simulink model "BeatDetection"  (R2015b)
settings: Solver=ode45  StartTime=0.0  StopTime=inf  RelTol=1e-3
undefined symbols (not defined in the file): dfilt, fdesignblkfcn, gcbh
libraries: simulink x13, dspmtrx3 x4, dsparch4 x3, dspvision x2, dspsnks4 x2, dspswit3 x1, dspxfrm3 x1, dspsigops x1
settings Model: Creator=Hegman  LastModifiedBy=Hegman
settings DataIOCC: SaveFormat=Array
settings DebuggingCC: SolverPrmCheckMsg=warning
settings HardwareCC: ProdBitPerPointer=32  ProdLargestAtomicFloat=None  ProdIntDivRoundTo=Undefined  ProdEndianess=Unspecified  ProdWordSize=32  ProdHWDeviceType=32-bit Generic
settings GRTTargetCC: GeneratePreprocessorConditionals=Disable all
settings ConfigComp: CovModelRefEnable=Off  CovSFcnEnable=off

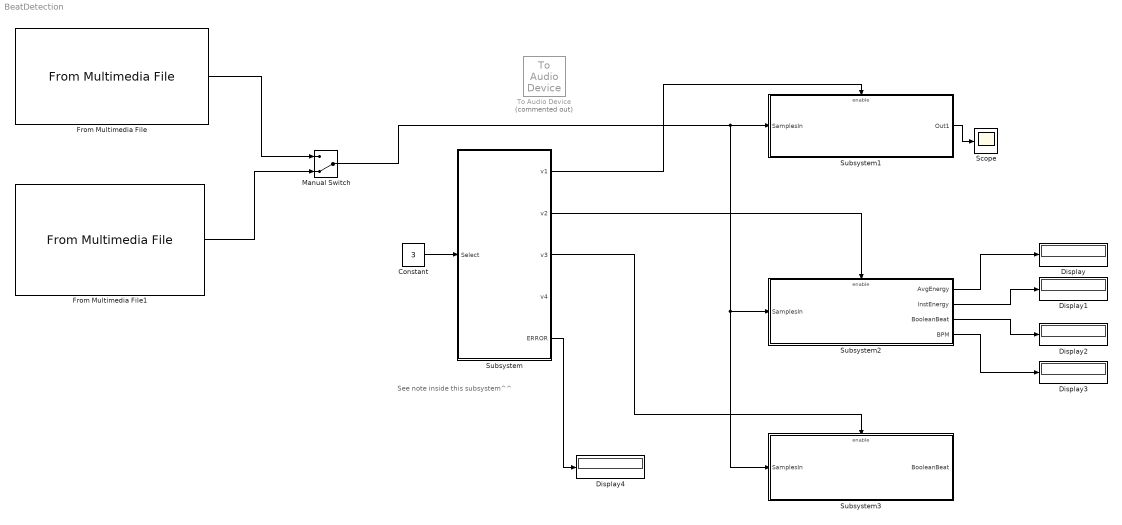
== system BeatDetection ==
  note: See note inside this subsystem^^
  Constant : Constant  Value=3
  Display{,1..4} (5 alike) : Display
  From Multimedia File : dspvision/From Multimedia File  inputFilename=C:\Users\Hegman\Desktop\bass.mp3  loop=on  numPlays=inf  outputStreams=Audio only  videoDataType=single  audioDataType=double  inheritSampleTime=on  userDefinedSampleTime=1/30  noAudioOutput=off  isIntensityVideo=off  fourcc=RGB  colorVideoFormat=Separate color signals  outputEOF=off  dataOrg=Column-major  audioFrameSize=1024  computeAudioFrameSize=off  outSamplingMode=Sample based
  From Multimedia File1 : dspvision/From Multimedia File  inputFilename=C:\Users\Hegman\Desktop\song.mp3  loop=on  numPlays=inf  outputStreams=Audio only  videoDataType=single  audioDataType=double  inheritSampleTime=on  userDefinedSampleTime=1/44  noAudioOutput=off  isIntensityVideo=off  fourcc=RGB  colorVideoFormat=Separate color signals  outputEOF=off  dataOrg=Column-major  audioFrameSize=1024  computeAudioFrameSize=off  outSamplingMode=Sample based
  Manual Switch : ManualSwitch  CurrentSetting=0
  Scope : Scope
  Subsystem : Subsystem
  Subsystem1 : Subsystem
  Subsystem2 : Subsystem
  Subsystem3 : Subsystem
  To Audio Device : dspsnks4/To Audio Device  Commented=on  deviceName=Default  inheritSampleRate=on  sampleRate=45056  deviceDatatype=Determine from input data type  autoBufferSize=on  bufferSize=4096  queueDuration=1.0  defaultOutputChannelMapping=on  outputChannelMapping=1:2  outputNumUnderrunSamples=off
  wires:
  Subsystem1/1(Out1) -> Scope/1
  Subsystem2/1(AvgEnergy) -> Display/1
  Subsystem2/2(InstEnergy) -> Display1/1
  Subsystem2/3(BooleanBeat) -> Display2/1
  Subsystem2/4(BPM) -> Display3/1
  Subsystem/1(v1) -> Subsystem1/Enable
  Subsystem/2(v2) -> Subsystem2/Enable
  Constant/1 -> Subsystem/1(Select)
  Subsystem/3(v3) -> Subsystem3/Enable
  Subsystem/5(ERROR) -> Display4/1
  From Multimedia File/1 -> Manual Switch/1
  From Multimedia File1/1 -> Manual Switch/2
  Manual Switch/1 -> Subsystem2/1(SamplesIn), Subsystem3/1(SamplesIn), Subsystem1/1(SamplesIn)

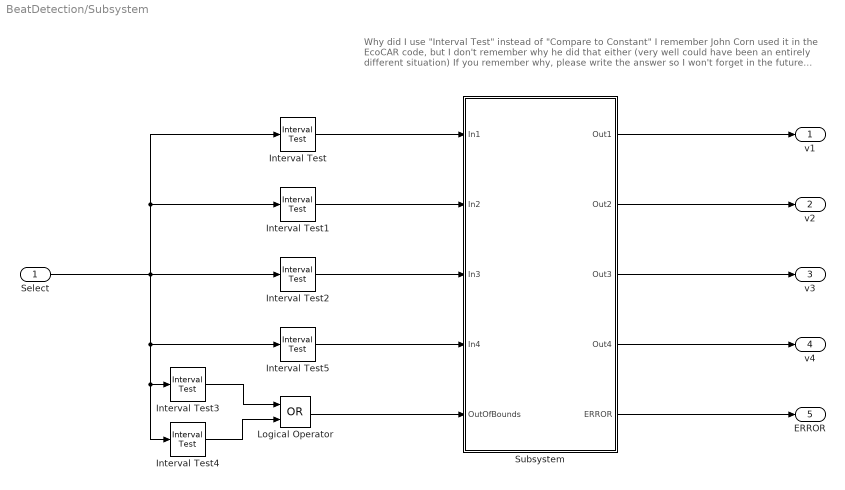
== system BeatDetection/Subsystem ==
  note: Why did I use "Interval Test" instead of "Compare to Constant"
      | I remember John Corn used it in the EcoCAR code, but I don't remember why he did that either (very well could have been an entirely different situation)
      | If you remember why, please write the answer so I won't forget in the future...
  Select : Inport
  Interval Test : simulink/Logic and Bit Operations/Interval Test  IntervalClosedRight=on  uplimit=1  IntervalClosedLeft=on  lowlimit=1  OutDataTypeStr=uint8
  Interval Test1 : simulink/Logic and Bit Operations/Interval Test  IntervalClosedRight=on  uplimit=2  IntervalClosedLeft=on  lowlimit=2  OutDataTypeStr=uint8
  Interval Test2 : simulink/Logic and Bit Operations/Interval Test  IntervalClosedRight=on  uplimit=3  IntervalClosedLeft=on  lowlimit=3  OutDataTypeStr=uint8
  Interval Test3 : simulink/Logic and Bit Operations/Interval Test  IntervalClosedRight=off  uplimit=1  IntervalClosedLeft=on  lowlimit=-inf  OutDataTypeStr=boolean
  Interval Test4 : simulink/Logic and Bit Operations/Interval Test  IntervalClosedRight=on  uplimit=inf  IntervalClosedLeft=off  lowlimit=3  OutDataTypeStr=boolean
  Interval Test5 : simulink/Logic and Bit Operations/Interval Test  IntervalClosedRight=on  uplimit=4  IntervalClosedLeft=on  lowlimit=4  OutDataTypeStr=uint8
  Logical Operator : Logic  Operator=OR  AllPortsSameDT=off
  Subsystem : Subsystem
  v1 : Outport
  v2 : Outport  Port=2
  v3 : Outport  Port=3
  v4 : Outport  Port=4
  ERROR : Outport  Port=5
  wires:
  Interval Test3/1 -> Logical Operator/1
  Interval Test4/1 -> Logical Operator/2
  Select/1 -> Interval Test/1, Interval Test1/1, Interval Test5/1, Interval Test4/1, Interval Test3/1, Interval Test2/1
  Interval Test1/1 -> Subsystem/2(In2)
  Interval Test2/1 -> Subsystem/3(In3)
  Logical Operator/1 -> Subsystem/5(OutOfBounds)
  Interval Test/1 -> Subsystem/1(In1)
  Subsystem/1(Out1) -> v1/1
  Subsystem/2(Out2) -> v2/1
  Subsystem/3(Out3) -> v3/1
  Subsystem/5(ERROR) -> ERROR/1
  Interval Test5/1 -> Subsystem/4(In4)
  Subsystem/4(Out4) -> v4/1

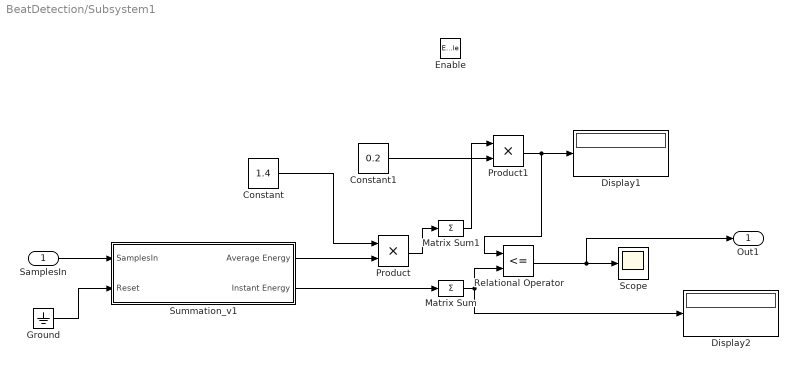
== system BeatDetection/Subsystem1 ==
  SamplesIn : Inport
  Enable : EnablePort
  Constant : Constant  Value=1.4
  Constant1 : Constant  Value=0.2
  Display1 : Display
  Display2 : Display
  Ground : Ground
  Matrix Sum : Sum  Inputs=+
  Matrix Sum1 : Sum  Inputs=+
  Product : Product
  Product1 : Product
  Relational Operator : RelationalOperator  Operator=<=  OutDataTypeStr=boolean
  Scope : Scope
  Summation_v1 : Subsystem
  Out1 : Outport
  wires:
  Summation_v1/1(Average Energy) -> Product/2
  Constant/1 -> Product/1
  Relational Operator/1 -> Out1/1, Scope/1
  Summation_v1/2(Instant Energy) -> Matrix Sum/1
  Matrix Sum/1 -> Display2/1, Relational Operator/2
  Product/1 -> Matrix Sum1/1
  Product1/1 -> Relational Operator/1, Display1/1
  Matrix Sum1/1 -> Product1/1
  Constant1/1 -> Product1/2
  SamplesIn/1 -> Summation_v1/1(SamplesIn)
  Ground/1 -> Summation_v1/2(Reset)

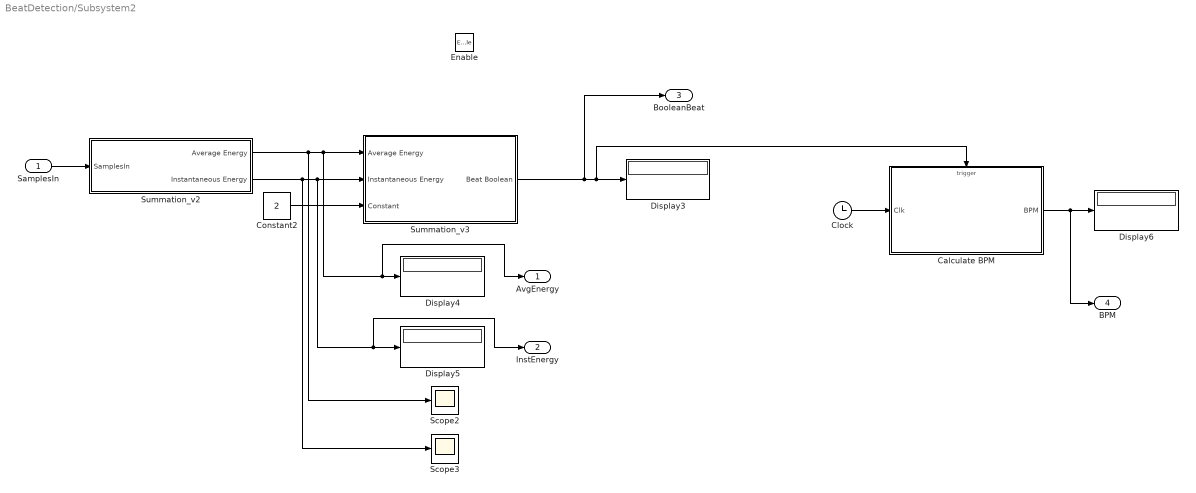
== system BeatDetection/Subsystem2 ==
  SamplesIn : Inport
  Enable : EnablePort
  Calculate BPM : Subsystem
  Clock : Clock
  Constant2 : Constant  Value=2
  Display{3..6} (4 alike) : Display
  Scope2 : Scope
  Scope3 : Scope
  Summation_v2 : Subsystem
  Summation_v3 : Subsystem
  AvgEnergy : Outport
  InstEnergy : Outport  Port=2
  BooleanBeat : Outport  Port=3
  BPM : Outport  Port=4
  wires:
  Summation_v2/1(Average Energy) -> Scope2/1, AvgEnergy/1, Display4/1, Summation_v3/1(Average Energy)
  Summation_v2/2(Instantaneous Energy) -> Scope3/1, InstEnergy/1, Display5/1, Summation_v3/2(Instantaneous Energy)
  Constant2/1 -> Summation_v3/3(Constant)
  Summation_v3/1(Beat Boolean) -> BooleanBeat/1, Calculate BPM/Trigger, Display3/1
  Clock/1 -> Calculate BPM/1(Clk)
  Calculate BPM/1(BPM) -> BPM/1, Display6/1
  SamplesIn/1 -> Summation_v2/1(SamplesIn)

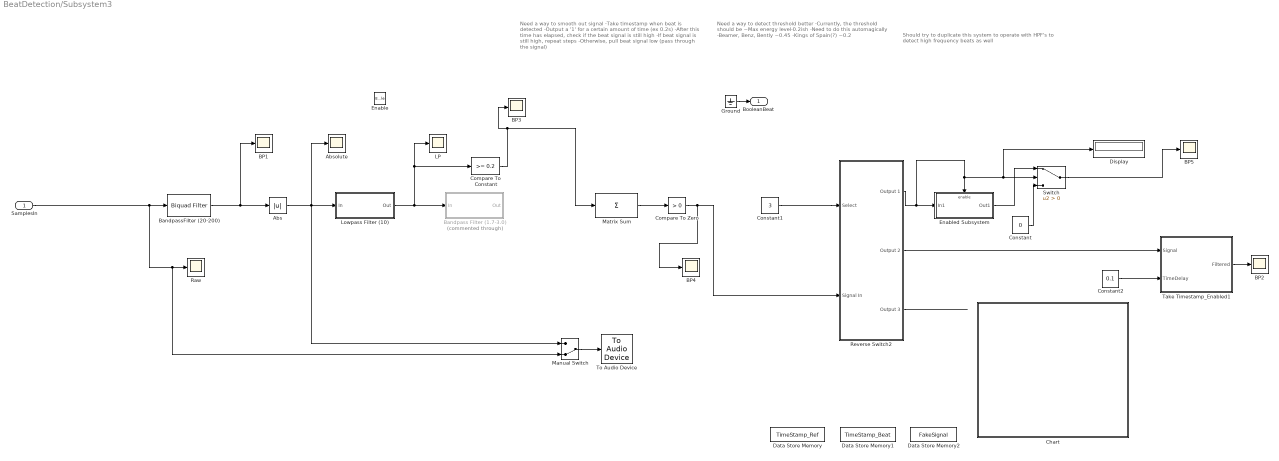
== system BeatDetection/Subsystem3 ==
  note: Need a way to smooth out signal
      | -Take timestamp when beat is detected
      | -Output a '1' for a certain amount of time (ex 0.2s)
      | -After this time has elapsed, check if the beat signal is still high
      | -If beat signal is still high, repeat steps
      | -Otherwise, pull beat signal low (pass through the signal)
  note: Need a way to detect threshold better
      | -Currently, the threshold should be ~Max energy level-0.2ish
      | -Need to do this automagically
      | -Beamer, Benz, Bently ~0.45
      | -Kings of Spain(?) ~0.2
  note: Should try to duplicate this system to operate with HPF's
      | to detect high frequency beats as well
  SamplesIn : Inport
  Enable : EnablePort
  Abs : Abs
  Absolute : Scope
  BP{1..5} (5 alike) : Scope
  Bandpass Filter (1.7-3.0) : Subsystem  Commented=through  DialogController=fdesignblkfcn  InitFcn=fdesignblkfcn(gcbh, {'InitFcn'});  mask(Bandpass Filter){}
      mask help: Design a bandpass filter
      settings: CopyFcn=fdesignblkfcn(gcbh, {'CopyFcn'});
      mask Help: helpview(mapfilelocation('dsp'), 'dspbandpassfilter');
      mask Display: disp('Bandpass');
  BandpassFilter (20-200) : dsparch4/Biquad Filter  Tag=BlockMethodSubSystem  IIRFiltStruct=Direct form II  CoeffSource=Specify via dialog  BiQuadCoeffs=[0.0031095318629756033 0 -0.0031095318629756033 1 -1.9981397557432883 0.99814821478936055;0.13570010317958014 0 -0.13570010317958014 1 -1.9940050318428257 0.9940167705198949;0.089106046740989542 0 -0.089106046740989542 1 -1.9816119239202097 0.98238370304407796;2 0 -2 1 -1.9589067705035481 0.95945538503128502]  a0Flag=Warning  IC=0  ICnum=0  ICden=0  InputProcessing=Columns as channels (frame based)  denAccumFracLength=30  denProdOutputFracLength=30  secondMemoryFracLength=15  roundingMode=Floor  overflowMode=off  ScaleValues=[5.1280917433920097e-06;1;1;1;67.812469673723953]  optimizeScaleValues=on  ScaleValueMode=Specify via input port (g)  scaleValueFracLength=14  FilterSource=Specify via dialog  FilterObject=dfilt.df2tsos([1 0.3 0.4],[1 0.1 0.2])
  Chart : Stateflow chart  TreatAsAtomicUnit=on
  Compare To Constant : simulink/Logic and Bit Operations/Compare To Constant  relop=>=  const=0.2  OutDataTypeStr=boolean
  Compare To Zero : simulink/Logic and Bit Operations/Compare To Zero  relop=>  OutDataTypeStr=uint8
  Constant : Constant  Value=0
  Constant1 : Constant  Value=3
  Constant2 : Constant  Value=0.1
  Data Store Memory : DataStoreMemory  DataStoreName=TimeStamp_Ref  ReadBeforeWriteMsg=warning  WriteAfterWriteMsg=warning  WriteAfterReadMsg=warning
  Data Store Memory1 : DataStoreMemory  DataStoreName=TimeStamp_Beat  ReadBeforeWriteMsg=warning  WriteAfterWriteMsg=warning  WriteAfterReadMsg=warning
  Data Store Memory2 : DataStoreMemory  DataStoreName=FakeSignal  ReadBeforeWriteMsg=warning  WriteAfterWriteMsg=warning  WriteAfterReadMsg=warning
  Display : Display
  Enabled Subsystem : Subsystem  TreatAsAtomicUnit=on
  Ground : Ground
  LP : Scope
  Lowpass Filter (10) : Subsystem  DialogController=fdesignblkfcn  InitFcn=fdesignblkfcn(gcbh, {'InitFcn'});  mask(Lowpass Filter){}
      mask help: Design a lowpass filter
      settings: CopyFcn=fdesignblkfcn(gcbh, {'CopyFcn'});
      mask Help: helpview(mapfilelocation('dsp'), 'dsplowpassfilter');
      mask Display: disp('Lowpass')
  Manual Switch : ManualSwitch  CurrentSetting=0
  Matrix Sum : Sum  Inputs=+
  Raw : Scope
  Reverse Switch2 : Subsystem
  Switch : Switch  Criteria=u2 > Threshold
  Take Timestamp_Enabled1 : Subsystem
  To Audio Device : dspsnks4/To Audio Device  deviceName=Default  inheritSampleRate=on  sampleRate=45056  deviceDatatype=Determine from input data type  autoBufferSize=on  bufferSize=4096  queueDuration=1.0  defaultOutputChannelMapping=on  outputChannelMapping=1:2  outputNumUnderrunSamples=off
  BooleanBeat : Outport
  wires:
  Ground/1 -> BooleanBeat/1
  SamplesIn/1 -> BandpassFilter (20-200)/1, Manual Switch/2, Raw/1
  BandpassFilter (20-200)/1 -> Abs/1, BP1/1
  Manual Switch/1 -> To Audio Device/1
  Abs/1 -> Manual Switch/1, Absolute/1, Lowpass Filter (10)/1(In)
  Lowpass Filter (10)/1(Out) -> Compare To Constant/1, LP/1, Bandpass Filter (1.7-3.0)/1(In)
  Compare To Constant/1 -> BP3/1, Matrix Sum/1
  Matrix Sum/1 -> Compare To Zero/1
  Compare To Zero/1 -> Reverse Switch2/2(Signal In), BP4/1
  Enabled Subsystem/1(Out1) -> Switch/1
  Constant/1 -> Switch/3
  Switch/1 -> BP5/1
  Reverse Switch2/1(Output 1) -> Display/1, Switch/2, Enabled Subsystem/Enable, Enabled Subsystem/1(In1)
  Reverse Switch2/2(Output 2) -> Take Timestamp_Enabled1/1(Signal)
  Constant1/1 -> Reverse Switch2/1(Select)
  Take Timestamp_Enabled1/1(Filtered) -> BP2/1
  Constant2/1 -> Take Timestamp_Enabled1/2(TimeDelay)
  Reverse Switch2/3(Output 3) -> ?

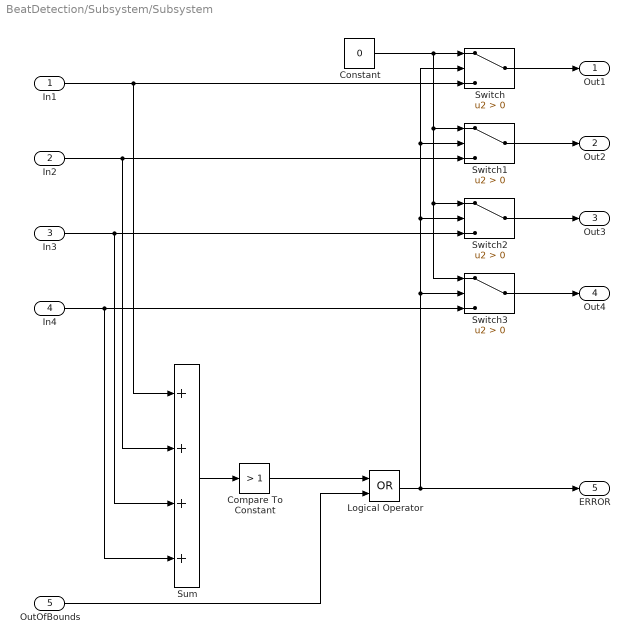
== system BeatDetection/Subsystem/Subsystem ==
  In1 : Inport
  In2 : Inport  Port=2
  In3 : Inport  Port=3
  In4 : Inport  Port=4
  OutOfBounds : Inport  Port=5
  Compare To Constant : simulink/Logic and Bit Operations/Compare To Constant  relop=>  const=1  OutDataTypeStr=boolean
  Constant : Constant  Value=0
  Logical Operator : Logic  Operator=OR  AllPortsSameDT=off  OutDataTypeStr=boolean
  Sum : Sum  Inputs=++++
  Switch{,1..3} (4 alike) : Switch  Criteria=u2 > Threshold
  Out1 : Outport
  Out2 : Outport  Port=2
  Out3 : Outport  Port=3
  Out4 : Outport  Port=4
  ERROR : Outport  Port=5
  wires:
  In1/1 -> Switch/3, Sum/1
  In2/1 -> Switch1/3, Sum/2
  In3/1 -> Switch2/3, Sum/3
  Sum/1 -> Compare To Constant/1
  OutOfBounds/1 -> Logical Operator/2
  Compare To Constant/1 -> Logical Operator/1
  Logical Operator/1 -> Switch3/2, Switch/2, Switch1/2, Switch2/2, ERROR/1
  Switch/1 -> Out1/1
  Switch1/1 -> Out2/1
  Switch2/1 -> Out3/1
  Constant/1 -> Switch2/1, Switch3/1, Switch1/1, Switch/1
  In4/1 -> Sum/4, Switch3/3
  Switch3/1 -> Out4/1

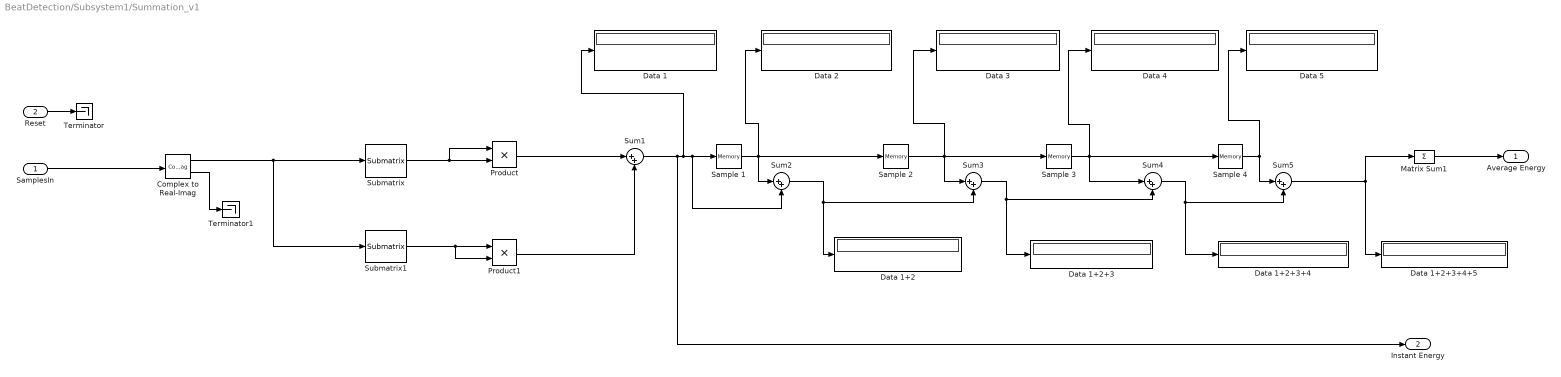
== system BeatDetection/Subsystem1/Summation_v1 ==
  SamplesIn : Inport
  Reset : Inport  Port=2
  Complex to Real-Imag : ComplexToRealImag
  Data {1..5} (5 alike) : Display
  Data 1+2 : Display
  Data 1+2+3 : Display
  Data 1+2+3+4 : Display
  Data 1+2+3+4+5 : Display
  Matrix Sum1 : Sum  Inputs=+
  Product : Product
  Product1 : Product
  Sample {1..4} (4 alike) : Memory
  Submatrix : dspmtrx3/Submatrix  RowSpan=Range of rows  RowStartMode=First  RowStartIndex=1  RowEndMode=Last  RowEndIndex=1  ColSpan=One column  ColStartMode=Index  ColStartIndex=1  ColEndMode=Last  ColEndIndex=1
  Submatrix1 : dspmtrx3/Submatrix  RowSpan=Range of rows  RowStartMode=First  RowStartIndex=1  RowEndMode=Last  RowEndIndex=1  ColSpan=One column  ColStartMode=Index  ColStartIndex=2  ColEndMode=Last  ColEndIndex=1
  Sum{1..5} (5 alike) : Sum  Inputs=|++
  Terminator : Terminator
  Terminator1 : Terminator
  Average Energy : Outport
  Instant Energy : Outport  Port=2
  wires:
  Submatrix1/1 -> Product1/2, Product1/1
  Submatrix/1 -> Product/2, Product/1
  Product/1 -> Sum1/1
  Product1/1 -> Sum1/2
  SamplesIn/1 -> Complex to Real-Imag/1
  Complex to Real-Imag/1 -> Submatrix1/1, Submatrix/1
  Complex to Real-Imag/2 -> Terminator1/1
  Sum1/1 -> Instant Energy/1, Sample 1/1, Sum2/2, Data 1/1
  Sample 1/1 -> Sum2/1, Sample 2/1, Data 2/1
  Sample 2/1 -> Sum3/1, Sample 3/1, Data 3/1
  Sample 3/1 -> Sum4/1, Sample 4/1, Data 4/1
  Sample 4/1 -> Sum5/1, Data 5/1
  Sum2/1 -> Sum3/2, Data 1+2/1
  Sum3/1 -> Sum4/2, Data 1+2+3/1
  Sum4/1 -> Sum5/2, Data 1+2+3+4/1
  Sum5/1 -> Data 1+2+3+4+5/1, Matrix Sum1/1
  Matrix Sum1/1 -> Average Energy/1
  Reset/1 -> Terminator/1

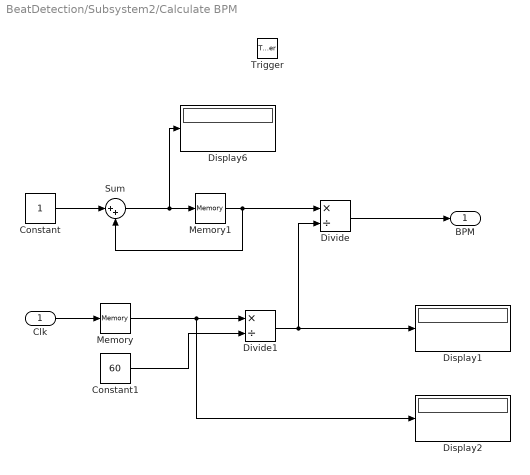
== system BeatDetection/Subsystem2/Calculate BPM ==
  Clk : Inport
  Trigger : TriggerPort  PortDimensions=1
  Constant : Constant
  Constant1 : Constant  Value=60
  Display1 : Display
  Display2 : Display
  Display6 : Display
  Divide : Product  Inputs=*/
  Divide1 : Product  Inputs=*/
  Memory : Memory  InheritSampleTime=on
  Memory1 : Memory  InheritSampleTime=on
  Sum : Sum  Inputs=|++
  BPM : Outport
  wires:
  Constant/1 -> Sum/1
  Sum/1 -> Display6/1, Memory1/1
  Memory1/1 -> Divide/1, Sum/2
  Clk/1 -> Memory/1
  Constant1/1 -> Divide1/2
  Memory/1 -> Display2/1, Divide1/1
  Divide1/1 -> Display1/1, Divide/2
  Divide/1 -> BPM/1

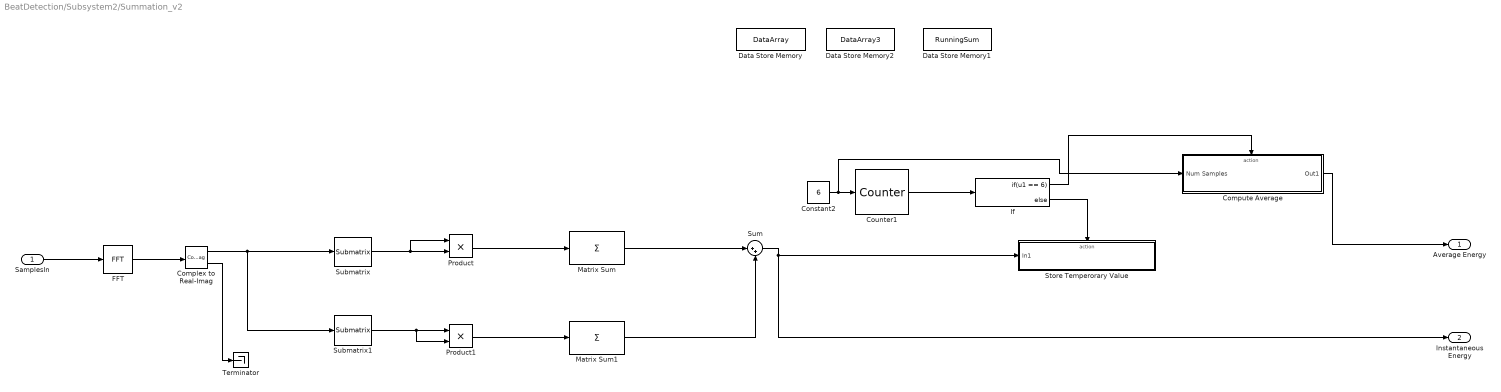
== system BeatDetection/Subsystem2/Summation_v2 ==
  SamplesIn : Inport
  Complex to Real-Imag : ComplexToRealImag
  Compute Average : Subsystem  TreatAsAtomicUnit=on
  Constant2 : Constant  Value=6  OutDataTypeStr=uint8
  Counter1 : dspswit3/Counter  Direction=Up  CountEvent=Free running  CounterSize=Specify via input port  MaxCount=43  InitialCount=0  Output=Count  HitValue=32  ResetInput=off  SamplesPerFrame=1  Ts=0.02321995464852607709750566893424  CntDtype=double  HitDtype=Logical
  Data Store Memory : DataStoreMemory  DataStoreName=DataArray  ReadBeforeWriteMsg=warning  WriteAfterWriteMsg=warning  WriteAfterReadMsg=warning  InitialValue=[0 0 0 0 0 0]
  Data Store Memory1 : DataStoreMemory  DataStoreName=RunningSum  ReadBeforeWriteMsg=warning  WriteAfterWriteMsg=warning  WriteAfterReadMsg=warning
  Data Store Memory2 : DataStoreMemory  DataStoreName=DataArray3  ReadBeforeWriteMsg=warning  WriteAfterWriteMsg=warning  WriteAfterReadMsg=warning  InitialValue=[0 0 0 0 0 0 0 0 0 0 0 0 0 0 0 0 0 0 0 0 0 0 0 0 0 0 0 0 0 0 0 0 0 0 0 0 0 0 0 0 0 0 0 0 0 0 0 0 0 0 0 0 0 0 0 0 0 0 0 0 0 0 0 0 0 0 0 0 0 0 0 0 0 0 0 0 0 0 0 0 0 0 0 0 0 0 0 0 0 0 0 0 0 0 0 0 0 0 0 0 0 0 0 0 0 0 0 0 0 0 0 0 0 0 0 0 0 0 0 0 0 0 0 0 0 0 0 0 0 0 0 0 0 0 0 0 0 0 0 0 0 0 0 0 0 0 0 0 0 0 0 0 0 0 0 0 0 0 0 0 0 0 0 0 0 0 0 0 0 0 0 0 0 0 0 0 0 0 0 0 0 0 0 0 0 0 0 0 0 0 0 0 0 0 0 0 0 0 0 0 0 0 0 0 0 0 0 0 0 0 0 0 0 0 0 0 0 0 0 0 0 0 0 0 0 0 0 0 0 0 0 0 0 0 0 0 0 0 0 0 0 0 0 0 0 0 0 0 0 0 0 0 0 0 0 0 0 0 0 0 0 0 0 0 0 0 0 0 0 0 0 0 0 0 0 0 0 0 0 0 0 0 0 0 0 0 0 0 0 0 0 0 0 0 0 0 0 0 0 0 0 0 0 0 0 0 0 0 0 0 0 0 0 0 0 0 0 0 0 0 0 0 0 0 0 0 0 0 0 0 0 0 0 0 0 0 0 0 0 0 0 0 0 0 0 0 0 0 0 0 0 0 0 0 0 0 0 0 0 0 0 0 0 0 0 0 0 0 0 0 0 0 0 0 0 0 0 0 0 0 0 0 0 0 0 0 0 0 0 0 0 0 0 0 0 0 0 0 0 0 0 0 0 0 0 0 0 0 0 0 0 0 0 0 0 0 0 0 0 0 0 0 0 0 0 0 0 0 0 0 0 0 0 0 0 0 0 0 0 0 0 0 0 0 0 0 0 0 0 0 0 0 0 0 0 0 0 0 0 0 0 0 0 0 0 0 0 0 0 0 0 0 0 0 0 0 0 0 0 0 0 0 0 0 0 0 0 0 0 0 0 0 0 0 0 0 0 0 0 0 0 0 0 0 0 0 0 0 0 0 0 0 0 0 0 0 0 0 0 0 0 0 0 0 0 0 0 0 0 0 0 0 0 0 0 0 0 0 0 0 0 0 0 0 0 0 0 0 0 0 0 0 0 0 0 0 0 0 0 0 0 0 0 0 0 0 0 0 0 0 0 0 0 0 0 0 0 0 0 0 0 0 0 0 0 0 0 0 0 0 0 0 0 0 0 0 0 0 0 0 0 0 0 0 0 0 0 0 0 0 0 0 0 0 0 0 0 0 0 0 0 0 0 0 0 0 0 0 0 0 0 0 0 0 0 0 0 0 0 0 0 0 0 0 0 0 0 0 0 0 0 0 0 0 0 0 0 0 0 0 0 0 0 0 0 0 0 0 0 0 0 0 0 0 0 0 0 0 0 0 0 0 0 0 0 0 0 0 0 0 0 0 0 0 0 0 0 0 0 0 0 0 0 0 0 0 0 0 0 0 0 0 0 0 0 0 0 0 0 0 0 0 0 0 0 0 0 0 0 0 0 0 0 0 0 0 0 0 0 0 0 0 0 0 0 0 0 0 0 0 0 0 0 0 0 0 0 0 0 0 0 0 0 0 0 0 0 0 0 0 0 0 0 0 0 0 0 0 0 0 0 0 0 0 0 0 0 0 0 0 0 0 0 0 0 0 0 0 0 0 0 0 0 0 0 0 0 0 0 0 0 0 0 0 0 0 0 0 0 0 0 0 0 0 0 0 0 0 0 0 0 0 0 0 0 0 0 0 0 0 0 0 0 0 0 0 0 0 0 0 0 0 0 0 0 0 0 0 0 0 0 0 0 0 0 0 0 0 0 0 0 0 0 0 0 0 0 0 0 0 0 0 0 0 0 0 0 0 0 0 0 0 0 0 0 0 0 0 0 0 0 0 0 0 0 0 0 0 0 0 0 0 0 0 0 0 0 0 0 0 0 0 0 0 0 0 0 0 0 0 0 0 0 0 0 0 0 0 0 0 0 0 0 0 0 0 0 0 0 0 0 0 0 0 0 0 0 0 0 0 0 0 0 0 0 0 0 0 0 0 0 0 0 0 0 0 0 0 0 0 0 0 0 0 0 0 0 0 0 0 0 0 0 0 0 0 0 0 0 0 0 0 0 0 0 0 0 0 0 0 0 0 0 0 0 0 0 0 0 0 0 0 0 0]
  FFT : dspxfrm3/FFT  FFTImplementation=Auto  CompMethod=Table lookup  TableOpt=NEW  TableOptActive=Speed  BitRevOrder=off  Normalize=off  InheritFFTLength=on  FFTLength=64  WrapInput=on  roundingMode=Floor  overflowMode=off  firstCoeffDataTypeStr=Inherit: Same word length as input  firstCoeffLastDataTypeStr=Inherit: Same word length as input  outputMin=[]  outputMax=[]
  If : If  IfExpression=u1 == 6
  Matrix Sum : Sum  Inputs=+
  Matrix Sum1 : Sum  Inputs=+
  Product : Product
  Product1 : Product
  Store Temperorary Value : Subsystem  TreatAsAtomicUnit=on
  Submatrix : dspmtrx3/Submatrix  RowSpan=Range of rows  RowStartMode=First  RowStartIndex=1  RowEndMode=Last  RowEndIndex=1  ColSpan=One column  ColStartMode=Index  ColStartIndex=1  ColEndMode=Last  ColEndIndex=1
  Submatrix1 : dspmtrx3/Submatrix  RowSpan=Range of rows  RowStartMode=First  RowStartIndex=1  RowEndMode=Last  RowEndIndex=1  ColSpan=One column  ColStartMode=Index  ColStartIndex=2  ColEndMode=Last  ColEndIndex=1
  Sum : Sum  Inputs=|++
  Terminator : Terminator
  Average Energy : Outport
  Instantaneous Energy : Outport  Port=2
  wires:
  Submatrix1/1 -> Product1/2, Product1/1
  Submatrix/1 -> Product/2, Product/1
  Product/1 -> Matrix Sum/1
  Product1/1 -> Matrix Sum1/1
  Matrix Sum/1 -> Sum/1
  Matrix Sum1/1 -> Sum/2
  Compute Average/1(Out1) -> Average Energy/1
  Constant2/1 -> Compute Average/1(Num Samples), Counter1/1
  Counter1/1 -> If/1
  If/1 -> Compute Average/Action
  Sum/1 -> Instantaneous Energy/1, Store Temperorary Value/1(In1)
  If/2 -> Store Temperorary Value/Action
  SamplesIn/1 -> FFT/1
  FFT/1 -> Complex to Real-Imag/1
  Complex to Real-Imag/1 -> Submatrix1/1, Submatrix/1
  Complex to Real-Imag/2 -> Terminator/1

== system BeatDetection/Subsystem2/Summation_v3 ==
  Average Energy : Inport
  Instantaneous Energy : Inport  Port=2
  Constant : Inport  Port=3
  Product : Product
  Relational Operator : RelationalOperator  Operator=<=  OutDataTypeStr=boolean
  Beat Boolean : Outport
  wires:
  Average Energy/1 -> Product/1
  Constant/1 -> Product/2
  Product/1 -> Relational Operator/1
  Instantaneous Energy/1 -> Relational Operator/2
  Relational Operator/1 -> Beat Boolean/1

== system BeatDetection/Subsystem3/Bandpass Filter (1.7-3.0) ==
  In : Inport
  Generated Filter Block : dsparch4/Biquad Filter  Tag=BlockMethodSubSystem  IIRFiltStruct=Direct form II  CoeffSource=Specify via dialog  BiQuadCoeffs=[5.4972901029509049e-05 0 -5.4972901029509049e-05 1 -1.9999520618723361 0.99995213446416487;0.00014448691002993394 0 -0.00014448691002993394 1 -1.9999059466356592 0.99990611089951908;9.0735971124424031e-05 0 -9.0735971124424031e-05 1 -1.999837449546598 0.99983750496372492;2 0 -2 1 -1.9998201282991981 0.99982028501520182]  a0Flag=Warning  IC=0  ICnum=0  ICden=0  InputProcessing=Columns as channels (frame based)  denAccumFracLength=30  denProdOutputFracLength=30  secondMemoryFracLength=15  roundingMode=Floor  overflowMode=off  ScaleValues=[7.259182877028536e-08;1;1;1;702.81183193528454]  optimizeScaleValues=off  ScaleValueMode=Specify via input port (g)  scaleValueFracLength=14  FilterSource=Specify via dialog  dfiltObjectName=dfilt.df2tsos([1 0.3 0.4],[1 0.1 0.2])
  Out : Outport
  wires:
  In/1 -> Generated Filter Block/1
  Generated Filter Block/1 -> Out/1

== system BeatDetection/Subsystem3/Enabled Subsystem ==
  In1 : Inport
  Enable : EnablePort
  Pulse Generator : DiscretePulseGenerator  PulseType=Time based  Period=0.4  PulseWidth=50
  Sample and Hold1 : dspsigops/Sample and Hold  trig=Either edge  initCond=0  latchinput=off
  Out1 : Outport
  wires:
  Sample and Hold1/1 -> Out1/1
  In1/1 -> Sample and Hold1/1
  Pulse Generator/1 -> Sample and Hold1/Trigger

== system BeatDetection/Subsystem3/Lowpass Filter (10) ==
  In : Inport
  Generated Filter Block : dsparch4/Biquad Filter  Tag=BlockMethodSubSystem  IIRFiltStruct=Direct form II  CoeffSource=Specify via dialog  BiQuadCoeffs=[3.3035044053868198e-07 6.6070088107736397e-07 3.3035044053868198e-07 1 -1.9976314897873875 0.99763351732213079;7.7829268025137561e-07 1.5565853605027512e-06 7.7829268025137561e-07 1 -1.9994422120745921 0.99944424144716315;5.0708276040372059e-07 1.0141655208074412e-06 5.0708276040372059e-07 1 -1.9972071092702939 0.99720913637430386;0.25000000910851183 0.50000001821702367 0.25000000910851183 1 -1.9984161174213928 0.99841814575250887]  a0Flag=Warning  IC=0  ICnum=0  ICden=0  InputProcessing=Columns as channels (frame based)  denAccumFracLength=30  denProdOutputFracLength=30  secondMemoryFracLength=15  roundingMode=Floor  overflowMode=off  ScaleValues=[2.0275347434317585e-06;1;1;1;1]  optimizeScaleValues=off  ScaleValueMode=Specify via input port (g)  scaleValueFracLength=14  FilterSource=Specify via dialog  FilterObject=dfilt.df2tsos([1 0.3 0.4],[1 0.1 0.2])
  Out : Outport
  wires:
  In/1 -> Generated Filter Block/1
  Generated Filter Block/1 -> Out/1

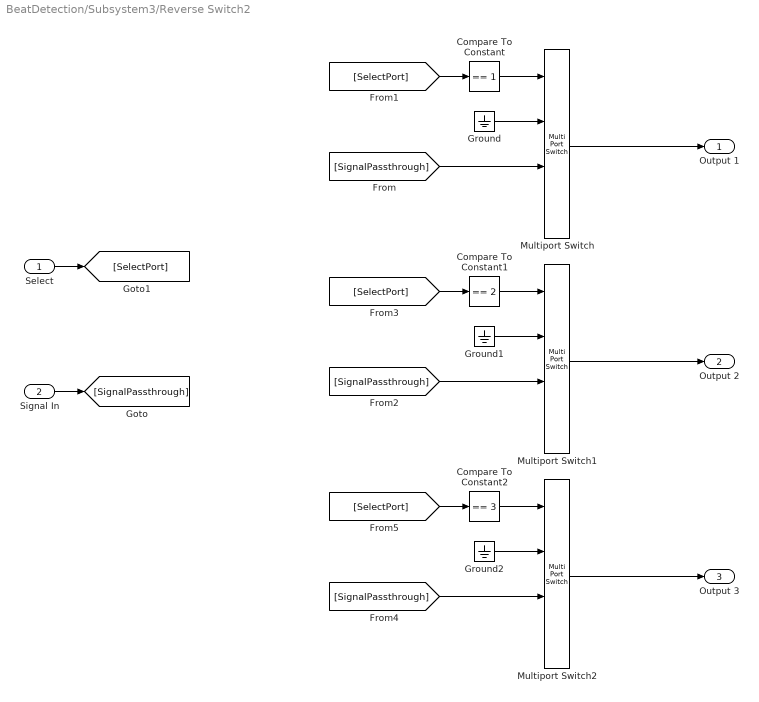
== system BeatDetection/Subsystem3/Reverse Switch2 ==
  Select : Inport
  Signal In : Inport  Port=2
  Compare To Constant : simulink/Logic and Bit Operations/Compare To Constant  relop===  const=1  OutDataTypeStr=uint8
  Compare To Constant1 : simulink/Logic and Bit Operations/Compare To Constant  relop===  const=2  OutDataTypeStr=uint8
  Compare To Constant2 : simulink/Logic and Bit Operations/Compare To Constant  relop===  const=3  OutDataTypeStr=uint8
  Ground : Ground
  Ground1 : Ground
  Ground2 : Ground
  Multiport Switch : MultiPortSwitch  DataPortOrder=Zero-based contiguous  Inputs=2  DataPortForDefault=Additional data port
  Multiport Switch1 : MultiPortSwitch  DataPortOrder=Zero-based contiguous  Inputs=2  DataPortForDefault=Additional data port
  Multiport Switch2 : MultiPortSwitch  DataPortOrder=Zero-based contiguous  Inputs=2  DataPortForDefault=Additional data port
  Output 1 : Outport
  Output 2 : Outport  Port=2
  Output 3 : Outport  Port=3
  wires:
  Compare To Constant/1 -> Multiport Switch/1
  Ground/1 -> Multiport Switch/2
  [SignalPassthrough] -> Multiport Switch/3
  Signal In/1 -> [SignalPassthrough]
  [SelectPort] -> Compare To Constant/1
  Compare To Constant1/1 -> Multiport Switch1/1
  Ground1/1 -> Multiport Switch1/2
  [SignalPassthrough] -> Multiport Switch1/3
  [SelectPort] -> Compare To Constant1/1
  Select/1 -> [SelectPort]
  Multiport Switch/1 -> Output 1/1
  Multiport Switch1/1 -> Output 2/1
  Compare To Constant2/1 -> Multiport Switch2/1
  Ground2/1 -> Multiport Switch2/2
  [SignalPassthrough] -> Multiport Switch2/3
  [SelectPort] -> Compare To Constant2/1
  Multiport Switch2/1 -> Output 3/1

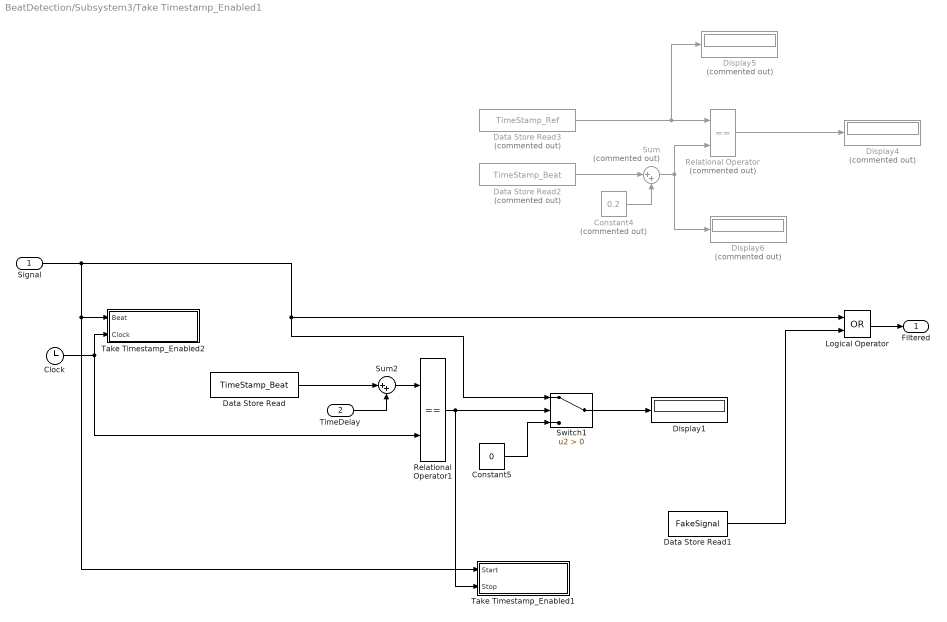
== system BeatDetection/Subsystem3/Take Timestamp_Enabled1 ==
  Signal : Inport
  TimeDelay : Inport  Port=2
  Clock : Clock
  Constant4 : Constant  Commented=on  Value=0.2
  Constant5 : Constant  Value=0
  Data Store Read : DataStoreRead  DataStoreName=TimeStamp_Beat  DataStoreElements=TimeStamp_Beat
  Data Store Read1 : DataStoreRead  DataStoreName=FakeSignal  DataStoreElements=FakeSignal
  Data Store Read2 : DataStoreRead  Commented=on  DataStoreName=TimeStamp_Beat  DataStoreElements=TimeStamp_Beat
  Data Store Read3 : DataStoreRead  Commented=on  DataStoreName=TimeStamp_Ref  DataStoreElements=TimeStamp_Ref
  Display1 : Display
  Display4 : Display  Commented=on
  Display5 : Display  Commented=on
  Display6 : Display  Commented=on
  Logical Operator : Logic  Operator=OR  AllPortsSameDT=off  OutDataTypeStr=boolean
  Relational Operator : RelationalOperator  Commented=on  Operator===  OutDataTypeStr=boolean
  Relational Operator1 : RelationalOperator  Operator===  OutDataTypeStr=boolean
  Sum : Sum  Commented=on  Inputs=|++
  Sum2 : Sum  Inputs=|++
  Switch1 : Switch  Criteria=u2 > Threshold
  Take Timestamp_Enabled1 : Subsystem
  Take Timestamp_Enabled2 : Subsystem
  Filtered : Outport
  wires:
  Data Store Read3/1 -> Display5/1, Relational Operator/1
  Constant4/1 -> Sum/2
  Sum/1 -> Relational Operator/2, Display6/1
  Relational Operator/1 -> Display4/1
  Data Store Read2/1 -> Sum/1
  Signal/1 -> Take Timestamp_Enabled1/1(Start), Take Timestamp_Enabled2/1(Beat), Logical Operator/1, Switch1/1
  Logical Operator/1 -> Filtered/1
  Sum2/1 -> Relational Operator1/1
  TimeDelay/1 -> Sum2/2
  Relational Operator1/1 -> Take Timestamp_Enabled1/2(Stop), Switch1/2
  Constant5/1 -> Switch1/3
  Switch1/1 -> Display1/1
  Clock/1 -> Relational Operator1/2, Take Timestamp_Enabled2/2(Clock)
  Data Store Read/1 -> Sum2/1
  Data Store Read1/1 -> Logical Operator/2

== system BeatDetection/Subsystem2/Summation_v2/Compute Average ==
  Num Samples : Inport
  Action Port : ActionPort  ActionType=then
  Constant1 : Constant  Commented=on  Value=-1
  Data Store Read : DataStoreRead  Commented=on  DataStoreName=RunningSum
  Data Store Read1 : DataStoreRead  DataStoreName=RunningSum
  Data Store Write : DataStoreWrite  Commented=on  DataStoreName=RunningSum
  Divide : Product  Inputs=*/
  Product : Product  Commented=on
  Sum1 : Sum  Commented=on  Inputs=|++
  Out1 : Outport
  wires:
  Num Samples/1 -> Divide/2
  Divide/1 -> Out1/1
  Product/1 -> Sum1/2
  Data Store Read/1 -> Sum1/1, Product/1
  Constant1/1 -> Product/2
  Sum1/1 -> Data Store Write/1
  Data Store Read1/1 -> Divide/1

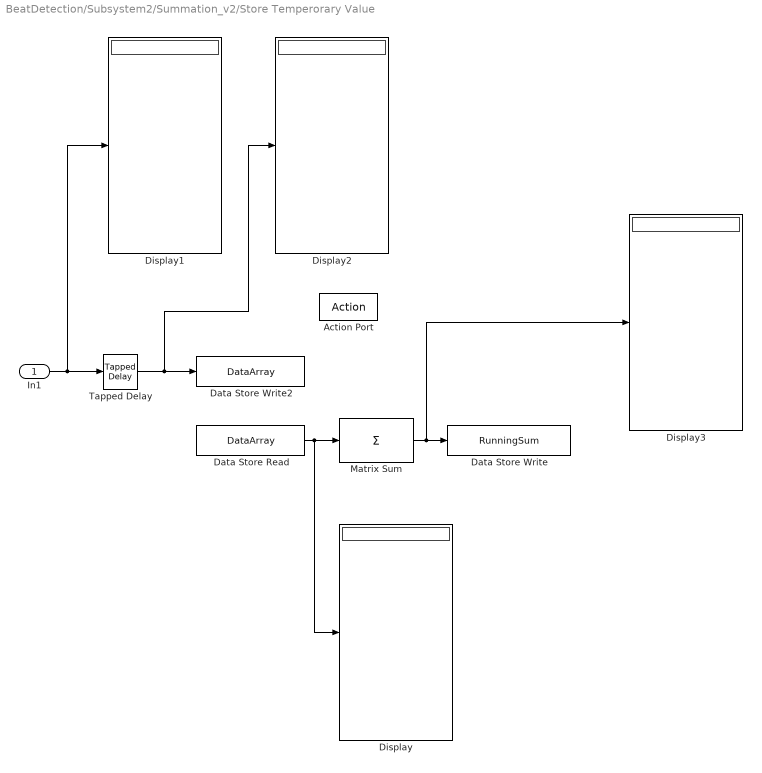
== system BeatDetection/Subsystem2/Summation_v2/Store Temperorary Value ==
  In1 : Inport
  Action Port : ActionPort  ActionType=else
  Data Store Read : DataStoreRead  DataStoreName=DataArray
  Data Store Write : DataStoreWrite  DialogController=Simulink.DDGSource  DataStoreName=RunningSum
  Data Store Write2 : DataStoreWrite  DialogController=Simulink.DDGSource  DataStoreName=DataArray
  Display{,1..3} (4 alike) : Display
  Matrix Sum : Sum  Inputs=+
  Tapped Delay : simulink/Discrete/Tapped Delay  vinit=0.0  samptime=-1  NumDelays=5  DelayOrder=Newest  includeCurrent=on
  wires:
  Data Store Read/1 -> Display/1, Matrix Sum/1
  Matrix Sum/1 -> Display3/1, Data Store Write/1
  In1/1 -> Display1/1, Tapped Delay/1
  Tapped Delay/1 -> Display2/1, Data Store Write2/1

== system BeatDetection/Subsystem3/Take Timestamp_Enabled1/Take Timestamp_Enabled1 ==
  Start : Inport
  Stop : Inport  Port=2
  If : If  IfExpression=u1 == 1  ShowElse=off
  If Action Subsystem : Subsystem  TreatAsAtomicUnit=on
  If Action Subsystem1 : Subsystem  TreatAsAtomicUnit=on
  If1 : If  IfExpression=u1 == 1  ShowElse=off
  wires:
  Start/1 -> If/1
  If/1 -> If Action Subsystem/Action
  Stop/1 -> If1/1
  If1/1 -> If Action Subsystem1/Action

== system BeatDetection/Subsystem3/Take Timestamp_Enabled1/Take Timestamp_Enabled2 ==
  Beat : Inport
  Clock : Inport  Port=2
  Data Store Read : DataStoreRead  DataStoreName=TimeStamp_Beat  DataStoreElements=TimeStamp_Beat
  Data Store Write : DataStoreWrite  DataStoreName=TimeStamp_Beat  DataStoreElements=TimeStamp_Beat
  Switch : Switch  Criteria=u2 > Threshold
  wires:
  Switch/1 -> Data Store Write/1
  Beat/1 -> Switch/2
  Data Store Read/1 -> Switch/3
  Clock/1 -> Switch/1

== system BeatDetection/Subsystem3/Take Timestamp_Enabled1/Take Timestamp_Enabled1/If Action Subsystem ==
  Action Port : ActionPort  ActionType=then
  Constant : Constant
  Data Store Write : DataStoreWrite  DataStoreName=FakeSignal  DataStoreElements=FakeSignal
  wires:
  Constant/1 -> Data Store Write/1

== system BeatDetection/Subsystem3/Take Timestamp_Enabled1/Take Timestamp_Enabled1/If Action Subsystem1 ==
  Action Port : ActionPort  ActionType=then
  Constant : Constant  Value=0
  Data Store Write : DataStoreWrite  DataStoreName=FakeSignal  DataStoreElements=FakeSignal
  wires:
  Constant/1 -> Data Store Write/1

== stateflow chart BeatDetection/Subsystem3/Chart ==
  state init
  state Beat_Output_On
    en: initTimeStamp = clock;
    beatOutput = 1
  state Beat_Output_Off
    en: beatOutput = 0
  (default) -> init
  Beat_Output_Off -> init
  init -> Beat_Output_On : [beatDetected == 1]
  (junction 9) -> Beat_Output_On [order 1] : [beatDetected == 1]
  Beat_Output_On -> (junction 9) : [clock > (initTimeStamp+timeBuffer)]
  (junction 9) -> Beat_Output_Off [order 2]
